simulink model "test_attitudeCtrl"  (R2015a)
settings: Solver=ode45  StartTime=0.0  StopTime=inf  RelTol=1e-3
libraries: CrazyFlie_lib x1
settings Model: Creator=rshum  LastModifiedBy=rshu

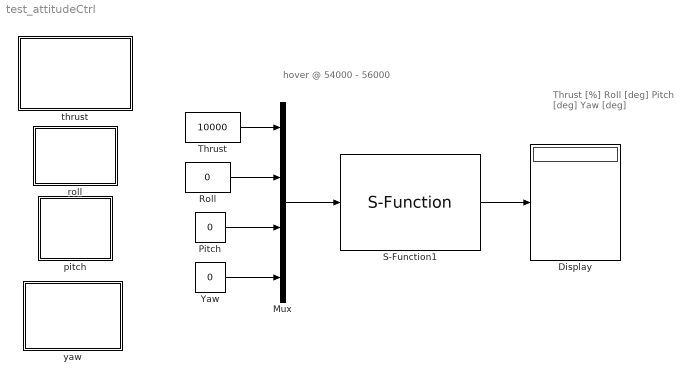
== system test_attitudeCtrl ==
  note: Thrust [%]
      | Roll [deg]
      | Pitch [deg]
      | Yaw [deg]
  note: hover @ 54000 - 56000
  Display : Display
  Mux : Mux
  Pitch : Constant  Value=0
  Roll : Constant  Value=0
  S-Function1 : CrazyFlie_lib/S-Function
  Thrust : Constant  Value=10000
  Yaw : Constant  Value=0
  pitch : Subsystem  DialogController=hmiCreateDDGDialog  IsWebBlock=on  mask(MathWorksWebBlock){webBlockId=95847192-24d1-4de3-ab52-ede6504f458f, webBlockType=continuousknob, ShowInLibBrowser=on, ShowInitialText=on, HMISrcModelName=test_attitude}
      mask prompts: webBlockId "WebBlock Id"; webBlockType "WebBlock Type"; HMISrcModelName "Source Model"
      mask Help: helpview([docroot '/mapfiles/simulink.map'], 'hmi_knob')
      mask Display:
      | if strcmp(get_param(bdroot(gcb),'BlockDiagramType'), 'library')
      |     image([(matlabroot) '/toolbox/simulink/hmi/icons/ContinuousKnob.png']);
      | end
  roll : Subsystem  DialogController=hmiCreateDDGDialog  IsWebBlock=on  mask(MathWorksWebBlock){webBlockId=88da0f21-1a35-48ca-bff8-4b546a046725, webBlockType=continuousknob, ShowInLibBrowser=on, ShowInitialText=on, HMISrcModelName=test_attitude}
      mask prompts: webBlockId "WebBlock Id"; webBlockType "WebBlock Type"; HMISrcModelName "Source Model"
      mask Help: helpview([docroot '/mapfiles/simulink.map'], 'hmi_knob')
      mask Display:
      | if strcmp(get_param(bdroot(gcb),'BlockDiagramType'), 'library')
      |     image([(matlabroot) '/toolbox/simulink/hmi/icons/ContinuousKnob.png']);
      | end
  "thrust " : Subsystem  DialogController=hmiCreateDDGDialog  IsWebBlock=on  mask(MathWorksWebBlock){webBlockId=fbd2dc25-91b7-4c0a-ac75-88661c3089d7, webBlockType=continuousknob, ShowInLibBrowser=on, ShowInitialText=on, HMISrcModelName=test_attitude}
      mask prompts: webBlockId "WebBlock Id"; webBlockType "WebBlock Type"; HMISrcModelName "Source Model"
      mask Help: helpview([docroot '/mapfiles/simulink.map'], 'hmi_knob')
      mask Display:
      | if strcmp(get_param(bdroot(gcb),'BlockDiagramType'), 'library')
      |     image([(matlabroot) '/toolbox/simulink/hmi/icons/ContinuousKnob.png']);
      | end
  yaw : Subsystem  DialogController=hmiCreateDDGDialog  IsWebBlock=on  mask(MathWorksWebBlock){webBlockId=0b0852f6-259a-485d-b41d-97be7ec8f41f, webBlockType=continuousknob, ShowInLibBrowser=on, ShowInitialText=on, HMISrcModelName=test_attitude}
      mask prompts: webBlockId "WebBlock Id"; webBlockType "WebBlock Type"; HMISrcModelName "Source Model"
      mask Help: helpview([docroot '/mapfiles/simulink.map'], 'hmi_knob')
      mask Display:
      | if strcmp(get_param(bdroot(gcb),'BlockDiagramType'), 'library')
      |     image([(matlabroot) '/toolbox/simulink/hmi/icons/ContinuousKnob.png']);
      | end
  wires:
  Mux/1 -> S-Function1/1
  Thrust/1 -> Mux/1
  Roll/1 -> Mux/2
  Pitch/1 -> Mux/3
  Yaw/1 -> Mux/4
  S-Function1/1 -> Display/1

== system test_attitudeCtrl/pitch ==

== system test_attitudeCtrl/roll ==

== system test_attitudeCtrl/thrust  ==

== system test_attitudeCtrl/yaw ==
